simulink model "MMR_IntegratedSimulation_FUZZYTEST"  (R2013a)
settings: Solver=ode3  StartTime=0.0  StopTime=Tstop  FixedStep=1e-2  RelTol=1e-3
values from neighbouring files (symbols this model uses):
  B = 0.0141    [parameters.m]
  Experiment = 2    [parameters.m]
  J = 0.0294    [parameters.m]
  Ke = 0.65    [parameters.m]
  Kt = 0.65    [parameters.m]
  L = 0.04    [parameters.m]
  Len = dis    (= 0)    [calc_len.m]    (also in parameters.m = 0.2)
  r = round(t/step + 1)    [TrajGen_MMR_FUZZYTEST.m]    (also in parameters.m = 0.045)
  R = 3.07    [parameters.m]
  R1_phi = 0.0    (= 0)    [parameters.m]
  R1_xi = 2.0    (= 2)    [parameters.m]
  R1_yi = 0.9    [parameters.m]
  R2_phi = 0.0    (= 0)    [parameters.m]
  R2_xi = -1.0    (= -1)    [parameters.m]
  R2_yi = 4.0    (= 4)    [parameters.m]
  R3_phi = 0.0    (= 0)    [parameters.m]
  R3_xi = 2.0    (= 2)    [parameters.m]
  R3_yi = -1.2    [parameters.m]
  Tstop = 210    [parameters.m]
libraries: simulink x9, fuzblock x6, dsparch4 x3
(part 2 of 2)

== system MMR_IntegratedSimulation_FUZZYTEST/Robot 2/Wheel Motor Controller/Left Motor Speed Controller and Motor Model/PMDC Motor Model ==
  V : Inport
  Tl : Inport  Port=2
  Constant : Constant  Value=2*pi
  Electrical : Fcn  Expr=-R/L*u(1)-Ke/L*u(2)+u(3)/L
  Integrator : Integrator
  Integrator1 : Integrator
  Integrator2 : Integrator
  Math Function : Math  Operator=rem  SaturateOnIntegerOverflow=on
  Mechanical : Fcn  Expr=-B/J*u(1)+Kt/J*u[2]-u(3)/J
  Mux : Mux  Inputs=3
  Mux1 : Mux  Inputs=3
  Theta : Outport
  w : Outport  Port=2
  I : Outport  Port=3
  wires:
  Constant/1 -> Math Function/2
  Integrator2/1 -> Math Function/1
  Math Function/1 -> Theta/1
  V/1 -> Mux1/3
  Integrator/1 -> Integrator2/1, Mux/1, Mux1/2, w/1
  Mux1/1 -> Electrical/1
  Electrical/1 -> Integrator1/1
  Integrator1/1 -> Mux/2, Mux1/1, I/1
  Mechanical/1 -> Integrator/1
  Tl/1 -> Mux/3
  Mux/1 -> Mechanical/1

== system MMR_IntegratedSimulation_FUZZYTEST/Robot 2/Wheel Motor Controller/Right Motor Speed Controller and Motor Model/PMDC Motor Model ==
  V : Inport
  Tl : Inport  Port=2
  Constant : Constant  Value=2*pi
  Electrical : Fcn  Expr=-R/L*u(1)-Ke/L*u(2)+u(3)/L
  Integrator : Integrator
  Integrator1 : Integrator
  Integrator2 : Integrator
  Math Function : Math  Operator=rem  SaturateOnIntegerOverflow=on
  Mechanical : Fcn  Expr=-B/J*u(1)+Kt/J*u[2]-u(3)/J
  Mux : Mux  Inputs=3
  Mux1 : Mux  Inputs=3
  Theta : Outport
  w : Outport  Port=2
  I : Outport  Port=3
  wires:
  Mux/1 -> Mechanical/1
  Tl/1 -> Mux/3
  Mechanical/1 -> Integrator/1
  Integrator1/1 -> I/1, Mux1/1, Mux/2
  Electrical/1 -> Integrator1/1
  Mux1/1 -> Electrical/1
  Integrator/1 -> w/1, Mux1/2, Mux/1, Integrator2/1
  V/1 -> Mux1/3
  Math Function/1 -> Theta/1
  Integrator2/1 -> Math Function/1
  Constant/1 -> Math Function/2

== system MMR_IntegratedSimulation_FUZZYTEST/Robot 3/Wheel Motor Controller/Left Motor Speed Controller and Motor Model/PMDC Motor Model ==
  V : Inport
  Tl : Inport  Port=2
  Constant : Constant  Value=2*pi
  Electrical : Fcn  Expr=-R/L*u(1)-Ke/L*u(2)+u(3)/L
  Integrator : Integrator
  Integrator1 : Integrator
  Integrator2 : Integrator
  Math Function : Math  Operator=rem  SaturateOnIntegerOverflow=on
  Mechanical : Fcn  Expr=-B/J*u(1)+Kt/J*u[2]-u(3)/J
  Mux : Mux  Inputs=3
  Mux1 : Mux  Inputs=3
  Theta : Outport
  w : Outport  Port=2
  I : Outport  Port=3
  wires:
  Constant/1 -> Math Function/2
  Integrator2/1 -> Math Function/1
  Math Function/1 -> Theta/1
  V/1 -> Mux1/3
  Integrator/1 -> Integrator2/1, Mux/1, Mux1/2, w/1
  Mux1/1 -> Electrical/1
  Electrical/1 -> Integrator1/1
  Integrator1/1 -> Mux/2, Mux1/1, I/1
  Mechanical/1 -> Integrator/1
  Tl/1 -> Mux/3
  Mux/1 -> Mechanical/1

== system MMR_IntegratedSimulation_FUZZYTEST/Robot 3/Wheel Motor Controller/Right Motor Speed Controller and Motor Model/PMDC Motor Model ==
  V : Inport
  Tl : Inport  Port=2
  Constant : Constant  Value=2*pi
  Electrical : Fcn  Expr=-R/L*u(1)-Ke/L*u(2)+u(3)/L
  Integrator : Integrator
  Integrator1 : Integrator
  Integrator2 : Integrator
  Math Function : Math  Operator=rem  SaturateOnIntegerOverflow=on
  Mechanical : Fcn  Expr=-B/J*u(1)+Kt/J*u[2]-u(3)/J
  Mux : Mux  Inputs=3
  Mux1 : Mux  Inputs=3
  Theta : Outport
  w : Outport  Port=2
  I : Outport  Port=3
  wires:
  Mux/1 -> Mechanical/1
  Tl/1 -> Mux/3
  Mechanical/1 -> Integrator/1
  Integrator1/1 -> I/1, Mux1/1, Mux/2
  Electrical/1 -> Integrator1/1
  Mux1/1 -> Electrical/1
  Integrator/1 -> w/1, Mux1/2, Mux/1, Integrator2/1
  V/1 -> Mux1/3
  Math Function/1 -> Theta/1
  Integrator2/1 -> Math Function/1
  Constant/1 -> Math Function/2
